simulink model "rct_helico1"  (R2020a)
settings: Solver=ode45  StartTime=0.0  StopTime=tspan(end)  RelTol=1e-3  EnableMultiTasking=on
model workspace (MAT data in the model file):
  A = [-0.0191  0.017  0.3839  -9.7924  -0.0008  -0.3371  0  0; 0.0136  -0.2994  0.0237  -0.5859  -0.0017  -0.0257  0.5374  0; 0.0405  -0.0026  -1.8394  0  0.0024  0.5281  0  -0.0015; 0  0  0.9985  0  0  0  0  0.0549; 0.001  -0.0017  -0.3381  0.0322  -0.0349  -0.4032  9.7777  0.1168; 0.013  0  -3.047  0  -0.229  -10.6199  0  -0.0333; 0  0  -0.0033  0  0  1  0  0.0598; 0.002  0.006  -0.5412  0  0.0039  -1.8554  0  -0.3487]
  B = [-10.3456  1.0793  0; -0.7293  0.0755  0; 27.09  -4.7239  -0.1857; 0  0  0; -1.082  -10.3713  4.7239; -27.2884  -156.4425  -1.069; 0  0  0; -4.8969  -27.9728  -12.9304]
  Cmeas = [0  0  0  1  0  0  0  0; 0  0  0  0  0  0  1  0; 0  0  0  0  0  0  0  1; 0  0  1  0  0  0  0  0; 0  0  0  0  0  1  0  0]
settings Model: FPTRunName=Active  Creator=The MathWorks, Inc.  LastModifiedBy=nikhil
settings DataIOCC: ExternalInput=[t__, u__]  SaveFormat=StructureWithTime
settings OptimizationCC: ExpressionDepthLimit=2147483647  LifeSpan=inf
settings DebuggingCC: UnderspecifiedInitializationDetection=Classic  MergeDetectMultiDrivingBlocksExec=none  FcnCallInpInsideContextMsg=warning  StateNameClashWarn=warning  SFUnexpectedBacktrackingDiag=warning  SFNoUnconditionalDefaultTransitionDiag=warning  SFExecutionAtInitializationDiag=none  ArithmeticOperatorsInVariantConditions=warning
settings HardwareCC: ProdBitPerPointer=32  ProdBitPerSizeT=32  ProdBitPerPtrDiffT=32  ProdLargestAtomicFloat=None  ProdIntDivRoundTo=Undefined  ProdEndianess=Unspecified  ProdWordSize=32  ProdHWDeviceType=32-bit Generic
settings ModelReferenceCC: PropagateSignalLabelsOutOfModel=off
settings SFSimCC: SimUseLocalCustomCode=off  CustomCodeUndefinedFunction=UseInterfaceOnly
settings RTWCC: RTWUseLocalCustomCode=off
settings CodeAppCC: StateflowObjectComments=on
settings GRTTargetCC: TargetLangStandard=C89/C90 (ANSI)  CombineOutputUpdateFcns=off  GRTInterface=on
settings ConfigComp: CovMetricSettings=dw  CovHtmlReporting=on  CovSaveCumulativeToWorkspaceVar=on  CovSaveSingleToWorkspaceVar=on  CovExternalEMLEnable=off

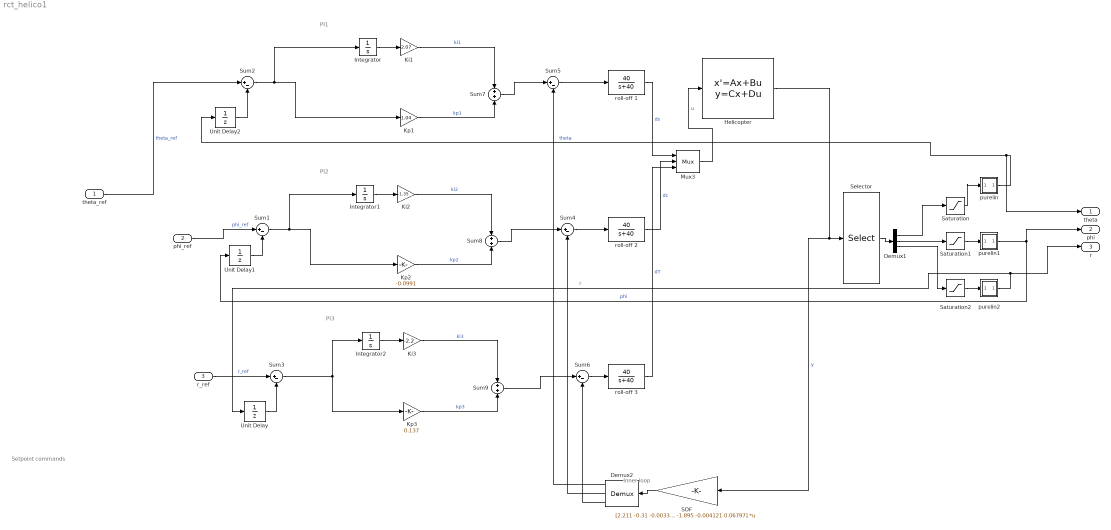
== system rct_helico1 ==
  note: PI3
  note: PI2
  note: PI1
  note: Setpoint
      | commands
  note: Inner loop
  theta_ref : Inport
  phi_ref : Inport  Port=2
  r_ref : Inport  Port=3
  Demux1 : Demux  Outputs=3
  Demux2 : Demux  Outputs=3
      settings: DisplayOption=none
  Helicopter : StateSpace  A=A  B=B  C=Cmeas  D=zeros(5,3)  InitialCondition=0
      mask Display: image('helico.jpg')
  Integrator : Integrator
  Integrator1 : Integrator
  Integrator2 : Integrator
  Ki1 : Gain  Gain=2.07
  Ki2 : Gain  Gain=-1.35
  Ki3 : Gain  Gain=-2.2
  Kp1 : Gain  Gain=1.04
  Kp2 : Gain  Gain=-0.0991
  Kp3 : Gain  Gain=0.137
  Mux3 : Mux  Inputs=3
      settings: DisplayOption=signals
  SOF : Gain  Gain=|  Multiplication=Matrix(K*u) (u vector)
      | [2.211 -0.31 -0.00336 0.7854 -0.01518;
      |   -0.1923  -1.291 0.0182  -0.08502 -0.1195;
      |  -0.01936  -0.01205 -1.895 -0.004121 0.06797]
  Saturation : Saturate
  Saturation1 : Saturate
  Saturation2 : Saturate
  Selector : Selector  InputPortWidth=5  IndexOptions=Index vector (dialog)  Indices=[1 2 3]  OutputSizes=3
  Sum{1..6} (6 alike) : Sum  Inputs=|+-
  Sum7 : Sum
  Sum8 : Sum
  Sum9 : Sum
  Unit Delay : UnitDelay  SampleTime=-1  HasFrameUpgradeWarning=on
  Unit Delay1 : UnitDelay  SampleTime=-1  HasFrameUpgradeWarning=on
  Unit Delay2 : UnitDelay  SampleTime=-1  HasFrameUpgradeWarning=on
  purelin : Subsystem
  purelin1 : Subsystem
  purelin2 : Subsystem
  roll-off 1 : TransferFcn  Numerator=[40]  Denominator=[1 40]
  roll-off 2 : TransferFcn  Numerator=[40]  Denominator=[1 40]
  roll-off 3 : TransferFcn  Numerator=[40]  Denominator=[1 40]
  theta : Outport
  phi : Outport  Port=2
  r : Outport  Port=3
  wires:
  Helicopter/1 -> SOF/1, Selector/1  "y"
  Mux3/1 -> Helicopter/1  "u"
  Sum4/1 -> roll-off 2/1
  roll-off 3/1 -> Mux3/3  "dT"
  roll-off 2/1 -> Mux3/2  "dc"
  roll-off 1/1 -> Mux3/1  "ds"
  phi_ref/1 -> Sum1/1  "phi_ref"
  theta_ref/1 -> Sum2/1  "theta_ref"
  r_ref/1 -> Sum3/1  "r_ref"
  Selector/1 -> Demux1/1
  Sum7/1 -> Sum5/1
  Sum5/1 -> roll-off 1/1
  SOF/1 -> Demux2/1
  Sum8/1 -> Sum4/1
  Sum9/1 -> Sum6/1
  Sum6/1 -> roll-off 3/1
  Demux2/1 -> Sum5/2
  Demux2/2 -> Sum4/2
  Demux2/3 -> Sum6/2
  Sum2/1 -> Kp1/1, Integrator/1
  Kp1/1 -> Sum7/2  "kp1"
  Ki1/1 -> Sum7/1  "ki1"
  Integrator/1 -> Ki1/1
  Ki2/1 -> Sum8/1  "ki2"
  Integrator1/1 -> Ki2/1
  Sum1/1 -> Kp2/1, Integrator1/1
  Kp2/1 -> Sum8/2  "kp2"
  Ki3/1 -> Sum9/1  "ki3"
  Integrator2/1 -> Ki3/1
  Sum3/1 -> Kp3/1, Integrator2/1
  Kp3/1 -> Sum9/2  "kp3"
  purelin/1(a) -> theta/1, Unit Delay2/1  "theta"
  purelin1/1(a) -> phi/1, Unit Delay1/1  "phi"
  purelin2/1(a) -> Unit Delay/1, r/1  "r"
  Unit Delay2/1 -> Sum2/2
  Unit Delay1/1 -> Sum1/2
  Unit Delay/1 -> Sum3/2
  Saturation1/1 -> purelin1/1(n)
  Saturation/1 -> purelin/1(n)
  Saturation2/1 -> purelin2/1(n)
  Demux1/1 -> Saturation/1
  Demux1/2 -> Saturation1/1
  Demux1/3 -> Saturation2/1

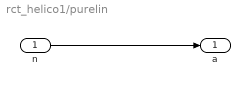
== system rct_helico1/purelin ==
  n : Inport
  a : Outport
  wires:
  n/1 -> a/1

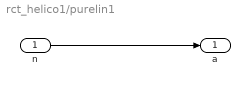
== system rct_helico1/purelin1 ==
  n : Inport
  a : Outport
  wires:
  n/1 -> a/1

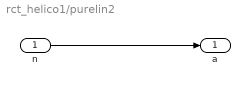
== system rct_helico1/purelin2 ==
  n : Inport
  a : Outport
  wires:
  n/1 -> a/1
